simulink model "pt8612_pll_detailed"  (Simulink 5.0)
settings: Solver=ode45  StartTime=0.0  StopTime=10.0  MaxStep=1/fpll/20  RelTol=1e-9  AbsTol=1e-12
values from neighbouring files (symbols this model uses):
  A = [[-1/Cp*(1/Rs+1/Rp) 1/Cp/Rs] ... (first row only)    [pt8612_analog_pll_init.m]    (also in pt8612_analog_pll_init_2.m = [[-1/C1/Ri     1/C1/Ri          0   ])
  B = [1/Cp 0].'    [pt8612_analog_pll_init.m]    (also in pt8612_analog_pll_init_2.m = [1/C1 0 0].')
  C = 680e-9    (= 6.8e-07)    [DPLL_init_2.m]    (also in pt8612_analog_pll_init.m = [1 0]; pt8612_analog_pll_init_2.m = [0 1 0]; pt8612_dpll_fpga_init.m; pt8612_dpll_fpga_init_2.m)
  fpll = fin/Ndec1    (= 296703.296703)    [DPLL_init_2.m]    (also in pt8612_analog_pll_init.m; pt8612_analog_pll_init_2.m; pt8612_dpll_fpga_init.m = 74175.8241758)
  fvcxo = 148.5e6/1.001    (= 148351648.352)    [DPLL_init_2.m]    (also in pt8612_analog_pll_init.m; pt8612_analog_pll_init_2.m; pt8612_dpll_fpga_init.m; pt8612_dpll_fpga_init_2.m = 148500000)
  Kvcxo = 90e-6    (= 9e-05)    [DPLL_init_2.m]    (also in pt8612_analog_pll_init.m; pt8612_analog_pll_init_2.m; pt8612_dpll_fpga_init.m; pt8612_dpll_fpga_init_2.m)
  Ri = 100e3    (= 100000)    [pt8612_analog_pll_init.m]    (also in pt8612_analog_pll_init_2.m)
  Vcc = 3.3    [DPLL_init_2.m]    (also in pt8612_analog_pll_init.m; pt8612_analog_pll_init_2.m; pt8612_dpll_fpga_init.m = 2.5; pt8612_dpll_fpga_init_2.m = 2.5)
  Vvcxo0 = 1.25    [DPLL_init_2.m]    (also in pt8612_analog_pll_init.m; pt8612_analog_pll_init_2.m; pt8612_dpll_fpga_init.m; pt8612_dpll_fpga_init_2.m)
libraries: simulink x4
settings Model: LastModifiedBy=thh

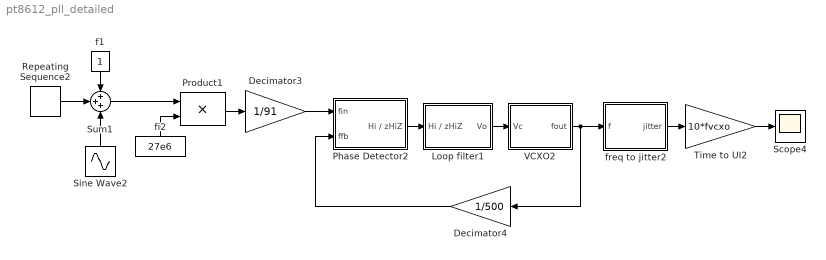
== system pt8612_pll_detailed ==
  Decimator3 : Gain  Gain=1/91  SaturateOnIntegerOverflow=on
  Decimator4 : Gain  Orientation=left  Gain=1/500  SaturateOnIntegerOverflow=on
  Loop filter1 : Subsystem
  Phase Detector2 : Subsystem
  Product1 : Product  SaturateOnIntegerOverflow=on
  Repeating Sequence2 : simulink/Sources/Repeating Sequence  rep_seq_t=[0 50 50 100]  rep_seq_y=[-1 -1 1 1]*0e-6
  Scope4 : Scope
      settings: TimeRange=10  YMin=3.9  YMax=6.1
  Sine Wave2 : Sin  Orientation=up  Amplitude=0e-6  SampleTime=0
  Sum1 : Sum  Inputs=+++  SaturateOnIntegerOverflow=on
  Time to UI2 : Gain  Gain=10*fvcxo  SaturateOnIntegerOverflow=on
  VCXO2 : Subsystem
  f1 : Constant  Orientation=down
  fi2 : Constant  Orientation=up  Value=27e6
  freq to jitter2 : Subsystem
  wires:
  freq to jitter2/1(jitter) -> Time to UI2/1
  Time to UI2/1 -> Scope4/1
  Product1/1 -> Decimator3/1
  f1/1 -> Sum1/1
  Sum1/1 -> Product1/1
  Repeating Sequence2/1 -> Sum1/2
  fi2/1 -> Product1/2
  Sine Wave2/1 -> Sum1/3
  Decimator3/1 -> Phase Detector2/1(fin)
  Phase Detector2/1(Hi / zHiZ) -> Loop filter1/1(Hi / zHiZ)
  Loop filter1/1(Vo) -> VCXO2/1(Vc)
  VCXO2/1(fout) -> Decimator4/1, freq to jitter2/1(f)
  Decimator4/1 -> Phase Detector2/2(ffb)

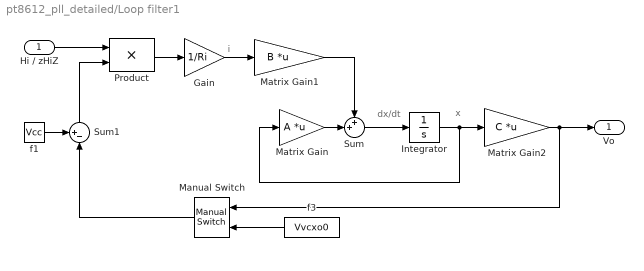
== system pt8612_pll_detailed/Loop filter1 ==
  note: i
  note: dx/dt
  note: x
  Hi / zHiZ : Inport
  Gain : Gain  Gain=1/Ri  SaturateOnIntegerOverflow=on
  Integrator : Integrator  InitialCondition=[1.25 1.25].'
  Manual Switch : simulink/Signal Routing/Manual Switch  Orientation=left  sw=1  action=0
  Matrix Gain : Gain  Gain=A  Multiplication=Matrix(K*u) (u vector)  SaturateOnIntegerOverflow=on
  Matrix Gain1 : Gain  Gain=B  Multiplication=Matrix(K*u)  SaturateOnIntegerOverflow=on
  Matrix Gain2 : Gain  Gain=C  Multiplication=Matrix(K*u) (u vector)  SaturateOnIntegerOverflow=on
  Product : Product  SaturateOnIntegerOverflow=on
  Sum : Sum  Inputs=++|  SaturateOnIntegerOverflow=on
  Sum1 : Sum  Orientation=up  Inputs=+-|  SaturateOnIntegerOverflow=on
  f1 : Constant  Value=Vcc
  f3 : Constant  Orientation=left  Value=Vvcxo0
  Vo : Outport
  wires:
  Hi / zHiZ/1 -> Product/1
  f1/1 -> Sum1/1
  Matrix Gain2/1 -> Vo/1, Manual Switch/1
  Sum1/1 -> Product/2
  Product/1 -> Gain/1
  Gain/1 -> Matrix Gain1/1
  Matrix Gain1/1 -> Sum/1
  Matrix Gain/1 -> Sum/2
  Sum/1 -> Integrator/1
  Integrator/1 -> Matrix Gain/1, Matrix Gain2/1
  Manual Switch/1 -> Sum1/2
  f3/1 -> Manual Switch/2

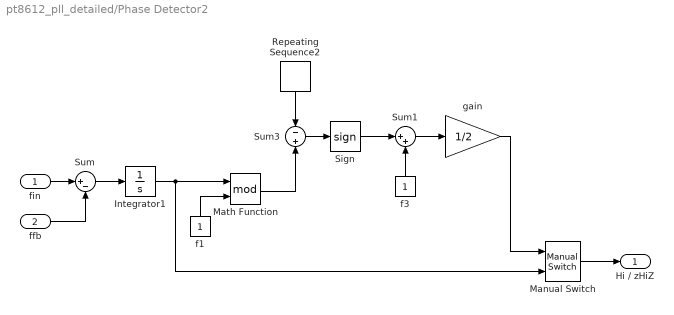
== system pt8612_pll_detailed/Phase Detector2 ==
  fin : Inport
  ffb : Inport  Port=2
  Integrator1 : Integrator  InitialCondition=0.062
  Manual Switch : simulink/Signal Routing/Manual Switch  sw=0  action=0
  Math Function : Math  Operator=mod
  Repeating Sequence2 : simulink/Sources/Repeating Sequence  Orientation=down  rep_seq_t=[0 1]/fpll  rep_seq_y=[0 1]
  Sign : Signum
  Sum : Sum  Inputs=|+-  SaturateOnIntegerOverflow=on
  Sum1 : Sum  Inputs=|++  SaturateOnIntegerOverflow=on
  Sum3 : Sum  Inputs=-|+  SaturateOnIntegerOverflow=on
  f1 : Constant  Orientation=up
  f3 : Constant  Orientation=up
  gain : Gain  Gain=1/2  SaturateOnIntegerOverflow=on
  Hi / zHiZ : Outport
  wires:
  Sum/1 -> Integrator1/1
  fin/1 -> Sum/1
  ffb/1 -> Sum/2
  Integrator1/1 -> Math Function/1, Manual Switch/2
  gain/1 -> Manual Switch/1
  f1/1 -> Math Function/2
  Math Function/1 -> Sum3/2
  Repeating Sequence2/1 -> Sum3/1
  f3/1 -> Sum1/2
  Sum3/1 -> Sign/1
  Sign/1 -> Sum1/1
  Sum1/1 -> gain/1
  Manual Switch/1 -> Hi / zHiZ/1

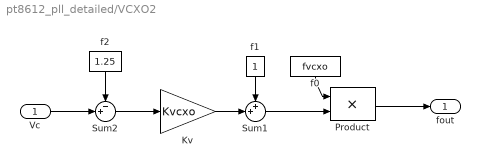
== system pt8612_pll_detailed/VCXO2 ==
  Vc : Inport
  Kv : Gain  Gain=Kvcxo  SaturateOnIntegerOverflow=on
  Product : Product  SaturateOnIntegerOverflow=on
  Sum1 : Sum  Inputs=++|  SaturateOnIntegerOverflow=on
  Sum2 : Sum  Inputs=-+|  SaturateOnIntegerOverflow=on
  f0 : Constant  Orientation=down  Value=fvcxo
  f1 : Constant  Orientation=down
  f2 : Constant  Orientation=down  Value=1.25
  fout : Outport
  wires:
  f0/1 -> Product/1
  f1/1 -> Sum1/1
  Sum1/1 -> Product/2
  Kv/1 -> Sum1/2
  Product/1 -> fout/1
  Sum2/1 -> Kv/1
  Vc/1 -> Sum2/2
  f2/1 -> Sum2/1

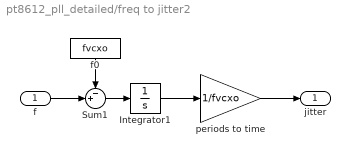
== system pt8612_pll_detailed/freq to jitter2 ==
  f : Inport
  Integrator1 : Integrator
  Sum1 : Sum  Inputs=-+|  SaturateOnIntegerOverflow=on
  f0 : Constant  Orientation=down  Value=fvcxo
  periods to time : Gain  Gain=1/fvcxo  SaturateOnIntegerOverflow=on
  jitter : Outport
  wires:
  Integrator1/1 -> periods to time/1
  Sum1/1 -> Integrator1/1
  f0/1 -> Sum1/1
  f/1 -> Sum1/2
  periods to time/1 -> jitter/1
